simulink subsystem "mesh_assembly"  (R2021a)
settings: Solver=VariableStepAuto  StartTime=0.0  StopTime=10.0  RelTol=1e-3
undefined symbols (not defined in the file): dnm, knm, X, Y, Z
libraries: sm_lib x110, mesh_assembly_library x15
(part 3 of 4)

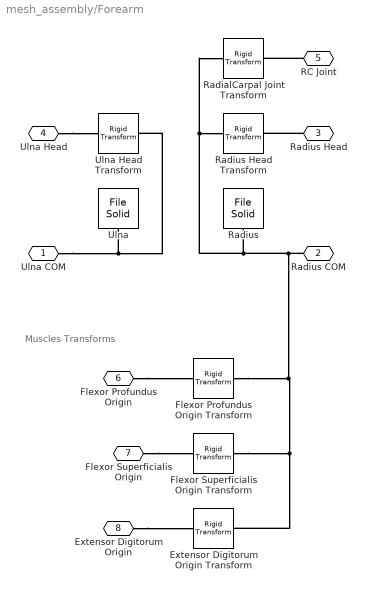
== system mesh_assembly/Forearm ==
  note: Muscles Transforms
  Extensor Digitorum Origin Transform : sm_lib/Frames and Transforms/Rigid Transform  TranslationMethod=Cartesian  TranslationStandardOffset=0  TranslationLengthUnit=m  TranslationStandardAxis=+Z  TranslationCartesianOffset=knm.radius.extensor_digitorum_origin(1,:)  TranslationROffset=0  TranslationROffsetUnits=m  TranslationZOffset=0  TranslationZOffsetUnits=m  TranslationThetaOffset=0  TranslationThetaOffsetUnits=deg  RotationMethod=RotationSequence  RotationAngleUnits=deg  RotationStandardAxis=+Z  RotationAngle=0.0  RotationArbitraryAxis=[0 0 1]  FollAlignAxisA=+X  BaseAlignAxisA=+Y  FollAlignAxisB=+Y  BaseAlignAxisB=+Z  RotationSequenceAxes=FollowerAxes  RotationSequence=XYZ  RotationSequenceAngles=knm.radius.extensor_digitorum_origin(2,:)  RotationSequenceAnglesUnits=deg  RotationMatrix=[1 0 0; 0 1 0; 0 0 1]
  Flexor Profundus Origin Transform : sm_lib/Frames and Transforms/Rigid Transform  TranslationMethod=Cartesian  TranslationStandardOffset=0  TranslationLengthUnit=m  TranslationStandardAxis=+Z  TranslationCartesianOffset=knm.radius.flexor_profundus_origin(1,:)  TranslationROffset=0  TranslationROffsetUnits=m  TranslationZOffset=0  TranslationZOffsetUnits=m  TranslationThetaOffset=0  TranslationThetaOffsetUnits=deg  RotationMethod=RotationSequence  RotationAngleUnits=deg  RotationStandardAxis=+Z  RotationAngle=0.0  RotationArbitraryAxis=[0 0 1]  FollAlignAxisA=+X  BaseAlignAxisA=+Y  FollAlignAxisB=+Y  BaseAlignAxisB=+Z  RotationSequenceAxes=FollowerAxes  RotationSequence=XYZ  RotationSequenceAngles=knm.radius.flexor_profundus_origin(2,:)  RotationSequenceAnglesUnits=deg  RotationMatrix=[1 0 0; 0 1 0; 0 0 1]
  Flexor Superficialis Origin Transform : sm_lib/Frames and Transforms/Rigid Transform  TranslationMethod=Cartesian  TranslationStandardOffset=0  TranslationLengthUnit=m  TranslationStandardAxis=+Z  TranslationCartesianOffset=knm.radius.flexor_superficialis_origin(1,:)  TranslationROffset=0  TranslationROffsetUnits=m  TranslationZOffset=0  TranslationZOffsetUnits=m  TranslationThetaOffset=0  TranslationThetaOffsetUnits=deg  RotationMethod=RotationSequence  RotationAngleUnits=deg  RotationStandardAxis=+Z  RotationAngle=0.0  RotationArbitraryAxis=[0 0 1]  FollAlignAxisA=+X  BaseAlignAxisA=+Y  FollAlignAxisB=+Y  BaseAlignAxisB=+Z  RotationSequenceAxes=FollowerAxes  RotationSequence=XYZ  RotationSequenceAngles=knm.radius.flexor_superficialis_origin(2,:)  RotationSequenceAnglesUnits=deg  RotationMatrix=[1 0 0; 0 1 0; 0 0 1]
  RadialCarpal Joint Transform : sm_lib/Frames and Transforms/Rigid Transform  TranslationMethod=Cartesian  TranslationStandardOffset=0  TranslationLengthUnit=m  TranslationStandardAxis=+Z  TranslationCartesianOffset=knm.radius.rc_joint_transform(1, :)  TranslationROffset=0  TranslationROffsetUnits=m  TranslationZOffset=0  TranslationZOffsetUnits=m  TranslationThetaOffset=0  TranslationThetaOffsetUnits=deg  RotationMethod=RotationSequence  RotationAngleUnits=deg  RotationStandardAxis=+Z  RotationAngle=0.0  RotationArbitraryAxis=[0 0 1]  FollAlignAxisA=+X  BaseAlignAxisA=+Y  FollAlignAxisB=+Y  BaseAlignAxisB=+Z  RotationSequenceAxes=FollowerAxes  RotationSequence=XYZ  RotationSequenceAngles=knm.radius.rc_joint_transform(2, :)  RotationSequenceAnglesUnits=deg  RotationMatrix=[1 0 0; 0 1 0; 0 0 1]
  Radius : sm_lib/Body Elements/File Solid  ExtGeomFileName=C:\Users\Daniel Adejumo\Documents\MATLAB\DARM\Geometry Models and FEA\Models\Skeleton Scan\Right Hand\Radius.obj  UnitType=Custom  ExtGeomFileUnits=mm  StepReaderType=HEX  ExportConvexHullGeometry=off  InertiaType=CalculateFromGeometry  Mass=1  MassUnits=kg  CenterOfMass=[0 0 0]  CenterOfMassUnits=m  MomentsOfInertia=[1 1 1]  MomentsOfInertiaUnits=kg*m^2  ProductsOfInertia=[0 0 0]  ProductsOfInertiaUnits=kg*m^2  BasedOnType=Density  Density=dnm.link_density  DensityUnits=kg/m^3  DoExposeReferenceFrame=on  SerializedFrames=<Frames><Frame><Id>Frame1</Id><Value><Name>COM</Name><Origin><Source>CenterOfMassFrame</Source><FeatureName></FeatureName></Origin><PrimaryAxis><DefinedDirection>+Z</DefinedDirection><Source>ReferenceFrame</Source><SourceDirection>-Z</SourceDirection><FeatureName></FeatureName></PrimaryAxis><SecondaryAxis><DefinedDirection>+X</DefinedDirection><Source>ReferenceFrame</Source><SourceDirection>-Y</SourceDirection><FeatureName></FeatureName></SecondaryAxis></Value></Frame></Frames>  GraphicType=FromGeometry  MarkerShape=Sphere  MarkerSize=10  GraphicVisPropType=SimpleVisualProperties  GraphicDiffuseColor=[0.5 0.5 0.5]  GraphicSpecularColor=[0.5 0.5 0.5 1.0]  GraphicAmbientColor=[0.15 0.15 0.15 1.0]  GraphicEmissiveColor=[0.0 0.0 0.0 1.0]  GraphicShininess=75  GraphicOpacity=1.0
  Radius Head Transform : sm_lib/Frames and Transforms/Rigid Transform  TranslationMethod=Cartesian  TranslationStandardOffset=0  TranslationLengthUnit=m  TranslationStandardAxis=+Z  TranslationCartesianOffset=knm.radius.head_transform(1, :)  TranslationROffset=0  TranslationROffsetUnits=m  TranslationZOffset=0  TranslationZOffsetUnits=m  TranslationThetaOffset=0  TranslationThetaOffsetUnits=deg  RotationMethod=RotationSequence  RotationAngleUnits=deg  RotationStandardAxis=+Z  RotationAngle=0.0  RotationArbitraryAxis=[0 0 1]  FollAlignAxisA=+X  BaseAlignAxisA=+Y  FollAlignAxisB=+Y  BaseAlignAxisB=+Z  RotationSequenceAxes=FollowerAxes  RotationSequence=XYZ  RotationSequenceAngles=knm.radius.head_transform(2, :)  RotationSequenceAnglesUnits=deg  RotationMatrix=[1 0 0; 0 1 0; 0 0 1]
  Ulna : sm_lib/Body Elements/File Solid  ExtGeomFileName=C:\Users\Daniel Adejumo\Documents\MATLAB\DARM\Geometry Models and FEA\Models\Skeleton Scan\Right Hand\Ulna.obj  UnitType=Custom  ExtGeomFileUnits=mm  StepReaderType=HEX  ExportConvexHullGeometry=off  InertiaType=CalculateFromGeometry  Mass=1  MassUnits=kg  CenterOfMass=[0 0 0]  CenterOfMassUnits=m  MomentsOfInertia=[1 1 1]  MomentsOfInertiaUnits=kg*m^2  ProductsOfInertia=[0 0 0]  ProductsOfInertiaUnits=kg*m^2  BasedOnType=Density  Density=dnm.link_density  DensityUnits=kg/m^3  DoExposeReferenceFrame=on  SerializedFrames=<Frames><Frame><Id>Frame1</Id><Value><Name>COM</Name><Origin><Source>CenterOfMassFrame</Source><FeatureName></FeatureName></Origin><PrimaryAxis><DefinedDirection>+Z</DefinedDirection><Source>ReferenceFrame</Source><SourceDirection>-Z</SourceDirection><FeatureName></FeatureName></PrimaryAxis><SecondaryAxis><DefinedDirection>+X</DefinedDirection><Source>ReferenceFrame</Source><SourceDirection>-Y</SourceDirection><FeatureName></FeatureName></SecondaryAxis></Value></Frame></Frames>  GraphicType=FromGeometry  MarkerShape=Sphere  MarkerSize=10  GraphicVisPropType=SimpleVisualProperties  GraphicDiffuseColor=[0.5 0.5 0.5]  GraphicSpecularColor=[0.5 0.5 0.5 1.0]  GraphicAmbientColor=[0.15 0.15 0.15 1.0]  GraphicEmissiveColor=[0.0 0.0 0.0 1.0]  GraphicShininess=75  GraphicOpacity=1.0
  Ulna Head Transform : sm_lib/Frames and Transforms/Rigid Transform  TranslationMethod=Cartesian  TranslationStandardOffset=0  TranslationLengthUnit=m  TranslationStandardAxis=+Z  TranslationCartesianOffset=knm.ulna.head_transform(1, :)  TranslationROffset=0  TranslationROffsetUnits=m  TranslationZOffset=0  TranslationZOffsetUnits=m  TranslationThetaOffset=0  TranslationThetaOffsetUnits=deg  RotationMethod=RotationSequence  RotationAngleUnits=deg  RotationStandardAxis=+Z  RotationAngle=0.0  RotationArbitraryAxis=[0 0 1]  FollAlignAxisA=+X  BaseAlignAxisA=+Y  FollAlignAxisB=+Y  BaseAlignAxisB=+Z  RotationSequenceAxes=FollowerAxes  RotationSequence=XYZ  RotationSequenceAngles=knm.ulna.head_transform(2, :)  RotationSequenceAnglesUnits=deg  RotationMatrix=[1 0 0; 0 1 0; 0 0 1]
  Ulna COM : PMIOPort  Side=Left
  Radius COM : PMIOPort  Port=2  Side=Left
  Radius Head : PMIOPort  Port=3  Side=Left
  Ulna Head : PMIOPort  Port=4  Side=Left
  RC Joint : PMIOPort  Port=5  Side=Right
  Flexor Profundus Origin : PMIOPort  Port=6  Side=Left
  Flexor Superficialis Origin : PMIOPort  Port=7  Side=Left
  Extensor Digitorum Origin : PMIOPort  Port=8  Side=Left
  connections:
  Flexor Profundus Origin/RConn1 -- Flexor Profundus Origin Transform/RConn1
  Extensor Digitorum Origin/RConn1 -- Extensor Digitorum Origin Transform/RConn1
  Flexor Superficialis Origin/RConn1 -- Flexor Superficialis Origin Transform/RConn1
  Flexor Profundus Origin Transform/LConn1 -- Flexor Superficialis Origin Transform/LConn1 -- Extensor Digitorum Origin Transform/LConn1 -- Radius COM/RConn1 -- RadialCarpal Joint Transform/LConn1 -- Radius Head Transform/LConn1 -- Radius/LConn1
  Ulna COM/RConn1 -- Ulna/LConn1 -- Ulna Head Transform/LConn1
  RC Joint/RConn1 -- RadialCarpal Joint Transform/RConn1
  Radius Head/RConn1 -- Radius Head Transform/RConn1
  Ulna Head/RConn1 -- Ulna Head Transform/RConn1

== system mesh_assembly/RC Primitive Joint ==
  Universal Joint : sm_lib/Joints/Universal Joint  JointMode=Normal  SenseConstraintForce=off  SenseConstraintForceX=off  SenseConstraintForceY=off  SenseConstraintForceZ=off  SenseConstraintTorque=off  SenseConstraintTorqueX=off  SenseConstraintTorqueY=off  SenseConstraintTorqueZ=off  SenseTotalForce=off  SenseTotalForceX=off  SenseTotalForceY=off  SenseTotalForceZ=off  SenseTotalTorque=off  SenseTotalTorqueX=off  SenseTotalTorqueY=off  SenseTotalTorqueZ=off  CompositeWrenchDir=FollowerOnBase  CompositeWrenchFrame=BaseFrame  RxEquilibriumPosition=0  RxEquilibriumPositionUnits=deg  RxSpringStiffness=stiffness  RxSpringStiffnessUnits=N*m/deg  RxDampingCoefficient=damping  RxDampingCoefficientUnits=N*m/(deg/s)  RxTorqueActuationMode=NoTorque  RxMotionActuationMode=ComputedMotion  RxSensePosition=off  RxSenseVelocity=off  RxSenseAcceleration=off  RxSenseTorqueForce=off  RxSenseLowerLimitTorqueForce=off  RxSenseUpperLimitTorqueForce=off  RxLowerLimitSpecify=on  RxLowerLimitBound=x_limits(1)  RxLowerLimitBoundUnits=deg  RxLowerLimitStiffness=1e4  RxLowerLimitStiffnessUnits=N*m/deg  RxLowerLimitDamping=10  RxLowerLimitDampingUnits=N*m/(deg/s)  RxLowerLimitTransitionRegionWidth=0.1  RxLowerLimitTransitionRegionWidthUnits=deg  RxUpperLimitSpecify=on  RxUpperLimitBound=x_limits(2)  RxUpperLimitBoundUnits=deg  RxUpperLimitStiffness=1e4  RxUpperLimitStiffnessUnits=N*m/deg  RxUpperLimitDamping=10  RxUpperLimitDampingUnits=N*m/(deg/s)  RxUpperLimitTransitionRegionWidth=0.1  RxUpperLimitTransitionRegionWidthUnits=deg  RxPositionTargetSpecify=on  RxPositionTargetPriority=High  RxPositionTargetValue=x_initial_position  RxPositionTargetValueUnits=deg  RxVelocityTargetSpecify=off  RxVelocityTargetPriority=High  RxVelocityTargetValue=0  RxVelocityTargetValueUnits=deg/s  RyEquilibriumPosition=0  RyEquilibriumPositionUnits=deg  RySpringStiffness=stiffness  RySpringStiffnessUnits=N*m/deg  RyDampingCoefficient=damping  RyDampingCoefficientUnits=N*m/(deg/s)  RyTorqueActuationMode=NoTorque  RyMotionActuationMode=ComputedMotion  RySensePosition=off  RySenseVelocity=off  RySenseAcceleration=off  RySenseTorqueForce=off  RySenseLowerLimitTorqueForce=off  RySenseUpperLimitTorqueForce=off  RyLowerLimitSpecify=on  RyLowerLimitBound=y_limits(1)  RyLowerLimitBoundUnits=deg  RyLowerLimitStiffness=1e4  RyLowerLimitStiffnessUnits=N*m/deg  RyLowerLimitDamping=10  RyLowerLimitDampingUnits=N*m/(deg/s)  RyLowerLimitTransitionRegionWidth=0.1  RyLowerLimitTransitionRegionWidthUnits=deg  RyUpperLimitSpecify=on  RyUpperLimitBound=y_limits(2)  RyUpperLimitBoundUnits=deg  RyUpperLimitStiffness=1e4  RyUpperLimitStiffnessUnits=N*m/deg  RyUpperLimitDamping=10  RyUpperLimitDampingUnits=N*m/(deg/s)  RyUpperLimitTransitionRegionWidth=0.1  RyUpperLimitTransitionRegionWidthUnits=deg  RyPositionTargetSpecify=on  RyPositionTargetPriority=High  RyPositionTargetValue=y_initial_position  RyPositionTargetValueUnits=deg  RyVelocityTargetSpecify=off  RyVelocityTargetPriority=High  RyVelocityTargetValue=0  RyVelocityTargetValueUnits=deg/s
  X Axis Viz Transform : sm_lib/Frames and Transforms/Rigid Transform  TranslationMethod=None  TranslationStandardOffset=0  TranslationLengthUnit=m  TranslationStandardAxis=+Z  TranslationCartesianOffset=[0 0 0]  TranslationROffset=0  TranslationROffsetUnits=m  TranslationZOffset=0  TranslationZOffsetUnits=m  TranslationThetaOffset=0  TranslationThetaOffsetUnits=deg  RotationMethod=AlignedAxes  RotationAngleUnits=deg  RotationStandardAxis=+Z  RotationAngle=0.0  RotationArbitraryAxis=[0 0 1]  FollAlignAxisA=+Z  BaseAlignAxisA=+X  FollAlignAxisB=+X  BaseAlignAxisB=+Z  RotationSequenceAxes=FollowerAxes  RotationSequence=XYX  RotationSequenceAngles=[0 0 0]  RotationSequenceAnglesUnits=deg  RotationMatrix=[1 0 0; 0 1 0; 0 0 1]
  X Viz Cylinder : sm_lib/Body Elements/Revolved Solid  GraphicAmbientColor=[0.15 0.15 0.15 1.0]  BasedOnType=Mass  CenterOfMass=[0 0 0]  CenterOfMassUnits=m  GraphicDiffuseColor=x_color  ExportConvexHullGeometry=off  Density=1000  DensityUnits=kg/m^3  DoExposeReferenceFrame=on  GraphicEmissiveColor=[0.0 0.0 0.0 1.0]  ExportEntireGeometry=off  SerializedFrames=<Frames/>  MarkerShape=Sphere  MarkerSize=10  GraphicType=FromGeometry  InertiaType=CalculateFromGeometry  Mass=0  MassUnits=kg  MomentsOfInertia=[1 1 1]  MomentsOfInertiaUnits=kg*m^2  GraphicOpacity=x_opacity  ProductsOfInertia=[0 0 0]  ProductsOfInertiaUnits=kg*m^2  RevolutionCrossSection=|  RevolutionCrossSectionUnits=m  RevolutionAngle=180  RevolutionAngleUnits=deg  RevolutionExtent=Full  GraphicShininess=75  GraphicSpecularColor=[0.5 0.5 0.5 1.0]  GraphicVisPropType=SimpleVisualProperties
      | [x_radius, x_length/2;
      |  x_radius, -x_length/2;
      |  x_radius+thickness, -x_length/2;
      |  x_radius+thickness, x_length/2]
  Y Axis Viz Transform : sm_lib/Frames and Transforms/Rigid Transform  TranslationMethod=None  TranslationStandardOffset=0  TranslationLengthUnit=m  TranslationStandardAxis=+Z  TranslationCartesianOffset=[0 0 0]  TranslationROffset=0  TranslationROffsetUnits=m  TranslationZOffset=0  TranslationZOffsetUnits=m  TranslationThetaOffset=0  TranslationThetaOffsetUnits=deg  RotationMethod=AlignedAxes  RotationAngleUnits=deg  RotationStandardAxis=+Z  RotationAngle=0.0  RotationArbitraryAxis=[0 0 1]  FollAlignAxisA=+Z  BaseAlignAxisA=+Y  FollAlignAxisB=+X  BaseAlignAxisB=+Z  RotationSequenceAxes=FollowerAxes  RotationSequence=XYX  RotationSequenceAngles=[0 0 0]  RotationSequenceAnglesUnits=deg  RotationMatrix=[1 0 0; 0 1 0; 0 0 1]
  Y Viz Cylinder : sm_lib/Body Elements/Revolved Solid  GraphicAmbientColor=[0.15 0.15 0.15 1.0]  BasedOnType=Mass  CenterOfMass=[0 0 0]  CenterOfMassUnits=m  GraphicDiffuseColor=y_color  ExportConvexHullGeometry=off  Density=1000  DensityUnits=kg/m^3  DoExposeReferenceFrame=on  GraphicEmissiveColor=[0.0 0.0 0.0 1.0]  ExportEntireGeometry=off  SerializedFrames=<Frames/>  MarkerShape=Sphere  MarkerSize=10  GraphicType=FromGeometry  InertiaType=CalculateFromGeometry  Mass=0  MassUnits=kg  MomentsOfInertia=[1 1 1]  MomentsOfInertiaUnits=kg*m^2  GraphicOpacity=y_opacity  ProductsOfInertia=[0 0 0]  ProductsOfInertiaUnits=kg*m^2  RevolutionCrossSection=|  RevolutionCrossSectionUnits=m  RevolutionAngle=180  RevolutionAngleUnits=deg  RevolutionExtent=Full  GraphicShininess=75  GraphicSpecularColor=[0.5 0.5 0.5 1.0]  GraphicVisPropType=SimpleVisualProperties
      | [y_radius, y_length/2;
      |  y_radius, -y_length/2;
      |  y_radius+thickness, -y_length/2;
      |  y_radius+thickness, y_length/2]
  F : PMIOPort  Side=Right
  B : PMIOPort  Port=2  Side=Left
  connections:
  Y Viz Cylinder/RConn1 -- Y Axis Viz Transform/RConn1
  X Axis Viz Transform/RConn1 -- X Viz Cylinder/RConn1
  Y Axis Viz Transform/LConn1 -- Universal Joint/RConn1 -- F/RConn1
  X Axis Viz Transform/LConn1 -- B/RConn1 -- Universal Joint/LConn1

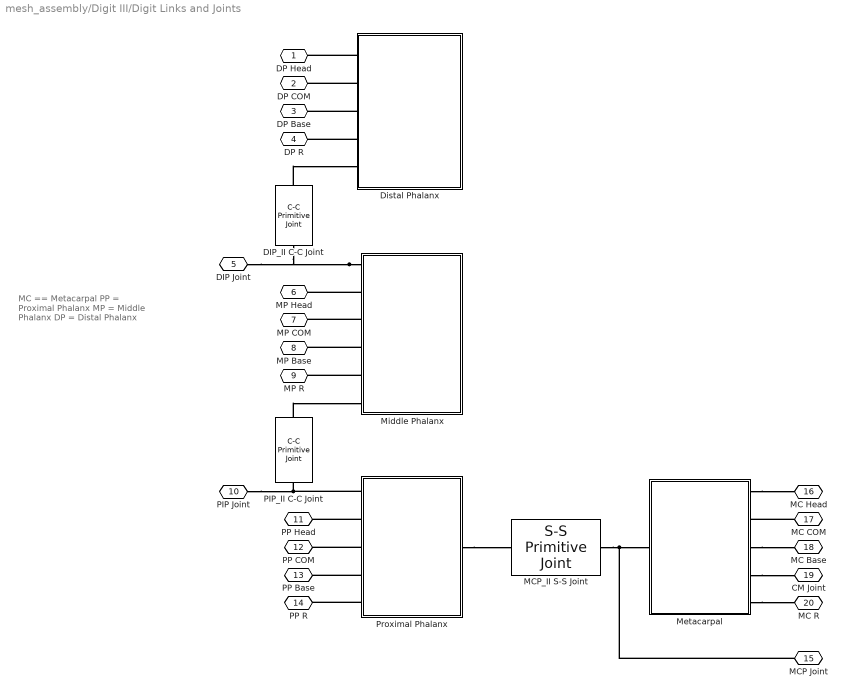
== system mesh_assembly/Digit III/Digit Links and Joints ==
  note: MC == Metacarpal
      | PP = Proximal Phalanx
      | MP = Middle Phalanx
      | DP = Distal Phalanx
  DIP_II C-C Joint : mesh_assembly_library/C-C Primitive Joint  stiffness=0  damping=0  lower_limit=-90  upper_limit=90  initial_position=0  radius=dip_viz_radius  length=dip_viz_length  thickness=dip_viz_thickness  color=dip_viz_color  opacity=dip_viz_opacity
  Distal Phalanx : Subsystem
  MCP_II S-S Joint : mesh_assembly_library/S-S Primitive Joint  stiffness=0  damping=0  x_limits=[-90 90]  y_limits=[-90 90]  x_initial_position=0  y_initial_position=0  radius=mcp_viz_radius  color=mcp_viz_color  opacity=mcp_viz_opacity
  Metacarpal : Subsystem
  Middle Phalanx : Subsystem
  PIP_II C-C Joint : mesh_assembly_library/C-C Primitive Joint  stiffness=0  damping=0  lower_limit=-90  upper_limit=90  initial_position=0  radius=pip_viz_radius  length=pip_viz_length  thickness=pip_viz_thickness  color=pip_viz_color  opacity=pip_viz_opacity
  Proximal Phalanx : Subsystem
  DP Head : PMIOPort  Side=Left
  DP COM : PMIOPort  Port=2  Side=Left
  DP Base : PMIOPort  Port=3  Side=Left
  DP R : PMIOPort  Port=4  Side=Left
  DIP Joint : PMIOPort  Port=5  Side=Left
  MP Head : PMIOPort  Port=6  Side=Left
  MP COM : PMIOPort  Port=7  Side=Left
  MP Base : PMIOPort  Port=8  Side=Left
  MP R : PMIOPort  Port=9  Side=Left
  PIP Joint : PMIOPort  Port=10  Side=Left
  PP Head : PMIOPort  Port=11  Side=Left
  PP COM : PMIOPort  Port=12  Side=Left
  PP Base : PMIOPort  Port=13  Side=Left
  PP R : PMIOPort  Port=14  Side=Left
  MCP Joint : PMIOPort  Port=15  Side=Left
  MC Head : PMIOPort  Port=16  Side=Left
  MC COM : PMIOPort  Port=17  Side=Left
  MC Base : PMIOPort  Port=18  Side=Left
  CM Joint : PMIOPort  Port=19  Side=Left
  MC R : PMIOPort  Port=20  Side=Left
  connections:
  Proximal Phalanx/LConn5 -- PP R/RConn1
  Proximal Phalanx/LConn4 -- PP Base/RConn1
  Proximal Phalanx/LConn2 -- PP Head/RConn1
  Distal Phalanx/LConn1 -- DP Head/RConn1
  Distal Phalanx/LConn2 -- DP COM/RConn1
  Metacarpal/RConn5 -- MC R/RConn1
  Metacarpal/RConn1 -- MC Head/RConn1
  Metacarpal/RConn4 -- CM Joint/RConn1
  Metacarpal/RConn3 -- MC Base/RConn1
  Middle Phalanx/LConn4 -- MP Base/RConn1
  Middle Phalanx/LConn2 -- MP Head/RConn1
  PIP_II C-C Joint/RConn1 -- Middle Phalanx/LConn6
  Distal Phalanx/LConn4 -- DP R/RConn1
  MCP Joint/RConn1 -- MCP_II S-S Joint/LConn1 -- Metacarpal/LConn1
  Middle Phalanx/LConn3 -- MP COM/RConn1
  Proximal Phalanx/LConn3 -- PP COM/RConn1
  Middle Phalanx/LConn1 -- DIP_II C-C Joint/LConn1 -- DIP Joint/RConn1
  Middle Phalanx/LConn5 -- MP R/RConn1
  Distal Phalanx/LConn3 -- DP Base/RConn1
  Proximal Phalanx/RConn1 -- MCP_II S-S Joint/RConn1
  PIP Joint/RConn1 -- Proximal Phalanx/LConn1 -- PIP_II C-C Joint/LConn1
  DIP_II C-C Joint/RConn1 -- Distal Phalanx/LConn5
  MC COM/RConn1 -- Metacarpal/RConn2

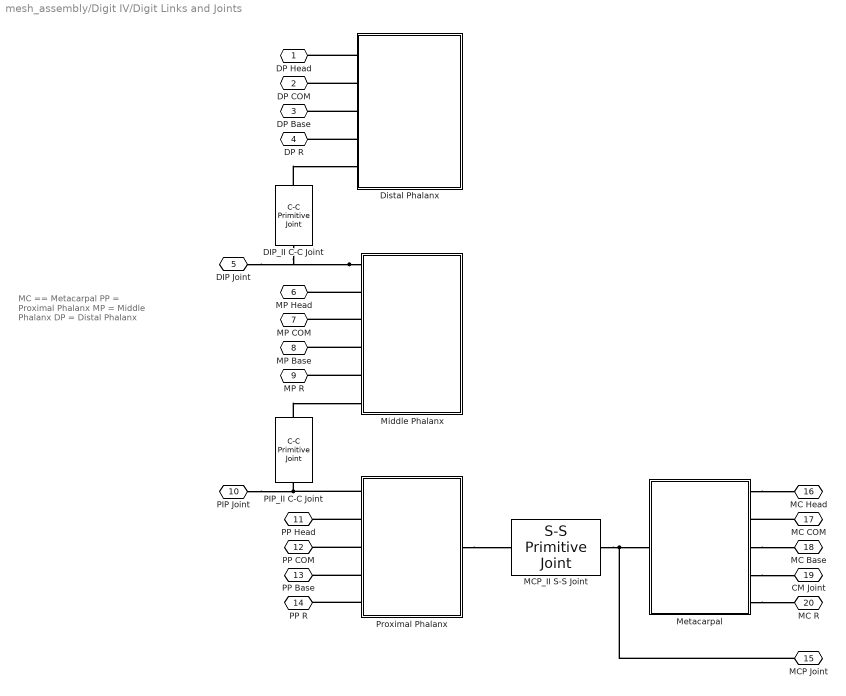
== system mesh_assembly/Digit IV/Digit Links and Joints ==
  note: MC == Metacarpal
      | PP = Proximal Phalanx
      | MP = Middle Phalanx
      | DP = Distal Phalanx
  DIP_II C-C Joint : mesh_assembly_library/C-C Primitive Joint  stiffness=0  damping=0  lower_limit=-90  upper_limit=90  initial_position=0  radius=dip_viz_radius  length=dip_viz_length  thickness=dip_viz_thickness  color=dip_viz_color  opacity=dip_viz_opacity
  Distal Phalanx : Subsystem
  MCP_II S-S Joint : mesh_assembly_library/S-S Primitive Joint  stiffness=0  damping=0  x_limits=[-90 90]  y_limits=[-90 90]  x_initial_position=0  y_initial_position=0  radius=mcp_viz_radius  color=mcp_viz_color  opacity=mcp_viz_opacity
  Metacarpal : Subsystem
  Middle Phalanx : Subsystem
  PIP_II C-C Joint : mesh_assembly_library/C-C Primitive Joint  stiffness=0  damping=0  lower_limit=-90  upper_limit=90  initial_position=0  radius=pip_viz_radius  length=pip_viz_length  thickness=pip_viz_thickness  color=pip_viz_color  opacity=pip_viz_opacity
  Proximal Phalanx : Subsystem
  DP Head : PMIOPort  Side=Left
  DP COM : PMIOPort  Port=2  Side=Left
  DP Base : PMIOPort  Port=3  Side=Left
  DP R : PMIOPort  Port=4  Side=Left
  DIP Joint : PMIOPort  Port=5  Side=Left
  MP Head : PMIOPort  Port=6  Side=Left
  MP COM : PMIOPort  Port=7  Side=Left
  MP Base : PMIOPort  Port=8  Side=Left
  MP R : PMIOPort  Port=9  Side=Left
  PIP Joint : PMIOPort  Port=10  Side=Left
  PP Head : PMIOPort  Port=11  Side=Left
  PP COM : PMIOPort  Port=12  Side=Left
  PP Base : PMIOPort  Port=13  Side=Left
  PP R : PMIOPort  Port=14  Side=Left
  MCP Joint : PMIOPort  Port=15  Side=Left
  MC Head : PMIOPort  Port=16  Side=Left
  MC COM : PMIOPort  Port=17  Side=Left
  MC Base : PMIOPort  Port=18  Side=Left
  CM Joint : PMIOPort  Port=19  Side=Left
  MC R : PMIOPort  Port=20  Side=Left
  connections:
  Proximal Phalanx/LConn5 -- PP R/RConn1
  Proximal Phalanx/LConn4 -- PP Base/RConn1
  Proximal Phalanx/LConn2 -- PP Head/RConn1
  Distal Phalanx/LConn1 -- DP Head/RConn1
  Distal Phalanx/LConn2 -- DP COM/RConn1
  Metacarpal/RConn5 -- MC R/RConn1
  Metacarpal/RConn1 -- MC Head/RConn1
  Metacarpal/RConn4 -- CM Joint/RConn1
  Metacarpal/RConn3 -- MC Base/RConn1
  Middle Phalanx/LConn4 -- MP Base/RConn1
  Middle Phalanx/LConn2 -- MP Head/RConn1
  PIP_II C-C Joint/RConn1 -- Middle Phalanx/LConn6
  Distal Phalanx/LConn4 -- DP R/RConn1
  MCP Joint/RConn1 -- MCP_II S-S Joint/LConn1 -- Metacarpal/LConn1
  Middle Phalanx/LConn3 -- MP COM/RConn1
  Proximal Phalanx/LConn3 -- PP COM/RConn1
  Middle Phalanx/LConn1 -- DIP_II C-C Joint/LConn1 -- DIP Joint/RConn1
  Middle Phalanx/LConn5 -- MP R/RConn1
  Distal Phalanx/LConn3 -- DP Base/RConn1
  Proximal Phalanx/RConn1 -- MCP_II S-S Joint/RConn1
  PIP Joint/RConn1 -- Proximal Phalanx/LConn1 -- PIP_II C-C Joint/LConn1
  DIP_II C-C Joint/RConn1 -- Distal Phalanx/LConn5
  MC COM/RConn1 -- Metacarpal/RConn2

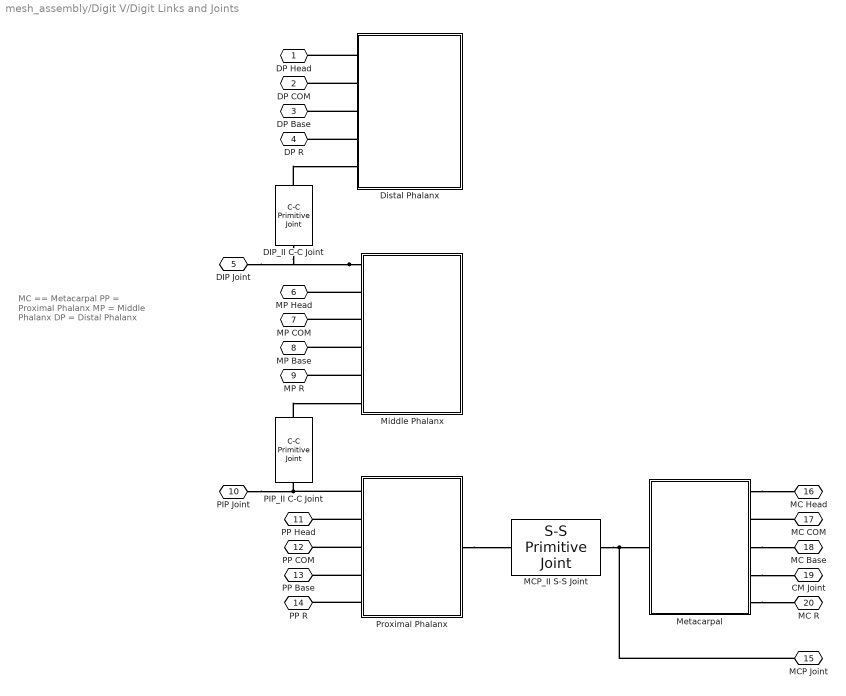
== system mesh_assembly/Digit V/Digit Links and Joints ==
  note: MC == Metacarpal
      | PP = Proximal Phalanx
      | MP = Middle Phalanx
      | DP = Distal Phalanx
  DIP_II C-C Joint : mesh_assembly_library/C-C Primitive Joint  stiffness=0  damping=0  lower_limit=-90  upper_limit=90  initial_position=0  radius=dip_viz_radius  length=dip_viz_length  thickness=dip_viz_thickness  color=dip_viz_color  opacity=dip_viz_opacity
  Distal Phalanx : Subsystem
  MCP_II S-S Joint : mesh_assembly_library/S-S Primitive Joint  stiffness=0  damping=0  x_limits=[-90 90]  y_limits=[-90 90]  x_initial_position=0  y_initial_position=0  radius=mcp_viz_radius  color=mcp_viz_color  opacity=mcp_viz_opacity
  Metacarpal : Subsystem
  Middle Phalanx : Subsystem
  PIP_II C-C Joint : mesh_assembly_library/C-C Primitive Joint  stiffness=0  damping=0  lower_limit=-90  upper_limit=90  initial_position=0  radius=pip_viz_radius  length=pip_viz_length  thickness=pip_viz_thickness  color=pip_viz_color  opacity=pip_viz_opacity
  Proximal Phalanx : Subsystem
  DP Head : PMIOPort  Side=Left
  DP COM : PMIOPort  Port=2  Side=Left
  DP Base : PMIOPort  Port=3  Side=Left
  DP R : PMIOPort  Port=4  Side=Left
  DIP Joint : PMIOPort  Port=5  Side=Left
  MP Head : PMIOPort  Port=6  Side=Left
  MP COM : PMIOPort  Port=7  Side=Left
  MP Base : PMIOPort  Port=8  Side=Left
  MP R : PMIOPort  Port=9  Side=Left
  PIP Joint : PMIOPort  Port=10  Side=Left
  PP Head : PMIOPort  Port=11  Side=Left
  PP COM : PMIOPort  Port=12  Side=Left
  PP Base : PMIOPort  Port=13  Side=Left
  PP R : PMIOPort  Port=14  Side=Left
  MCP Joint : PMIOPort  Port=15  Side=Left
  MC Head : PMIOPort  Port=16  Side=Left
  MC COM : PMIOPort  Port=17  Side=Left
  MC Base : PMIOPort  Port=18  Side=Left
  CM Joint : PMIOPort  Port=19  Side=Left
  MC R : PMIOPort  Port=20  Side=Left
  connections:
  Proximal Phalanx/LConn5 -- PP R/RConn1
  Proximal Phalanx/LConn4 -- PP Base/RConn1
  Proximal Phalanx/LConn2 -- PP Head/RConn1
  Distal Phalanx/LConn1 -- DP Head/RConn1
  Distal Phalanx/LConn2 -- DP COM/RConn1
  Metacarpal/RConn5 -- MC R/RConn1
  Metacarpal/RConn1 -- MC Head/RConn1
  Metacarpal/RConn4 -- CM Joint/RConn1
  Metacarpal/RConn3 -- MC Base/RConn1
  Middle Phalanx/LConn4 -- MP Base/RConn1
  Middle Phalanx/LConn2 -- MP Head/RConn1
  PIP_II C-C Joint/RConn1 -- Middle Phalanx/LConn6
  Distal Phalanx/LConn4 -- DP R/RConn1
  MCP Joint/RConn1 -- MCP_II S-S Joint/LConn1 -- Metacarpal/LConn1
  Middle Phalanx/LConn3 -- MP COM/RConn1
  Proximal Phalanx/LConn3 -- PP COM/RConn1
  Middle Phalanx/LConn1 -- DIP_II C-C Joint/LConn1 -- DIP Joint/RConn1
  Middle Phalanx/LConn5 -- MP R/RConn1
  Distal Phalanx/LConn3 -- DP Base/RConn1
  Proximal Phalanx/RConn1 -- MCP_II S-S Joint/RConn1
  PIP Joint/RConn1 -- Proximal Phalanx/LConn1 -- PIP_II C-C Joint/LConn1
  DIP_II C-C Joint/RConn1 -- Distal Phalanx/LConn5
  MC COM/RConn1 -- Metacarpal/RConn2

== system mesh_assembly/Digit III/Digit Links and Joints/Distal Phalanx ==
  Base Transform : sm_lib/Frames and Transforms/Rigid Transform  TranslationMethod=Cartesian  TranslationStandardOffset=0  TranslationLengthUnit=m  TranslationStandardAxis=+Z  TranslationCartesianOffset=distal_phalanx_base(1, :)  TranslationROffset=0  TranslationROffsetUnits=m  TranslationZOffset=0  TranslationZOffsetUnits=m  TranslationThetaOffset=0  TranslationThetaOffsetUnits=deg  RotationMethod=RotationSequence  RotationAngleUnits=deg  RotationStandardAxis=+Z  RotationAngle=0.0  RotationArbitraryAxis=[0 0 1]  FollAlignAxisA=+X  BaseAlignAxisA=+Y  FollAlignAxisB=+Y  BaseAlignAxisB=+Z  RotationSequenceAxes=FollowerAxes  RotationSequence=XYZ  RotationSequenceAngles=distal_phalanx_base(2, :)  RotationSequenceAnglesUnits=deg  RotationMatrix=[1 0 0; 0 1 0; 0 0 1]
  DIP Joint Transform : sm_lib/Frames and Transforms/Rigid Transform  TranslationMethod=Cartesian  TranslationStandardOffset=0  TranslationLengthUnit=m  TranslationStandardAxis=+Z  TranslationCartesianOffset=distal_phalanx_dip_joint(1, :)  TranslationROffset=0  TranslationROffsetUnits=m  TranslationZOffset=0  TranslationZOffsetUnits=m  TranslationThetaOffset=0  TranslationThetaOffsetUnits=deg  RotationMethod=RotationSequence  RotationAngleUnits=deg  RotationStandardAxis=+Z  RotationAngle=0.0  RotationArbitraryAxis=[0 0 1]  FollAlignAxisA=+X  BaseAlignAxisA=+Y  FollAlignAxisB=+Y  BaseAlignAxisB=+Z  RotationSequenceAxes=FollowerAxes  RotationSequence=XYZ  RotationSequenceAngles=distal_phalanx_dip_joint(2, :)  RotationSequenceAnglesUnits=deg  RotationMatrix=[1 0 0; 0 1 0; 0 0 1]
  Head Transform : sm_lib/Frames and Transforms/Rigid Transform  TranslationMethod=Cartesian  TranslationStandardOffset=0  TranslationLengthUnit=m  TranslationStandardAxis=+Z  TranslationCartesianOffset=distal_phalanx_head(1, :)  TranslationROffset=0  TranslationROffsetUnits=m  TranslationZOffset=0  TranslationZOffsetUnits=m  TranslationThetaOffset=0  TranslationThetaOffsetUnits=deg  RotationMethod=RotationSequence  RotationAngleUnits=deg  RotationStandardAxis=+Z  RotationAngle=0.0  RotationArbitraryAxis=[0 0 1]  FollAlignAxisA=+X  BaseAlignAxisA=+Y  FollAlignAxisB=+Y  BaseAlignAxisB=+Z  RotationSequenceAxes=FollowerAxes  RotationSequence=XYZ  RotationSequenceAngles=distal_phalanx_head(2, :)  RotationSequenceAnglesUnits=deg  RotationMatrix=[1 0 0; 0 1 0; 0 0 1]
  Rigid Body : sm_lib/Body Elements/File Solid  ExtGeomFileName=C:\Users\Daniel Adejumo\Documents\MATLAB\DARM\Geometry Models and FEA\Models\Skeleton Scan\Right Hand\Digit III\Distal Phalanx III.obj  UnitType=Custom  ExtGeomFileUnits=mm  StepReaderType=HEX  ExportConvexHullGeometry=off  InertiaType=CalculateFromGeometry  Mass=1  MassUnits=kg  CenterOfMass=[0 0 0]  CenterOfMassUnits=m  MomentsOfInertia=[1 1 1]  MomentsOfInertiaUnits=kg*m^2  ProductsOfInertia=[0 0 0]  ProductsOfInertiaUnits=kg*m^2  BasedOnType=Density  Density=links_density  DensityUnits=kg/m^3  DoExposeReferenceFrame=on  SerializedFrames=<Frames><Frame><Id>Frame1</Id><Value><Name>COM</Name><Origin><Source>CenterOfMassFrame</Source><FeatureName></FeatureName></Origin><PrimaryAxis><DefinedDirection>+Z</DefinedDirection><Source>ReferenceFrame</Source><SourceDirection>+X</SourceDirection><FeatureName></FeatureName></PrimaryAxis><SecondaryAxis><DefinedDirection>+X</DefinedDirection><Source>ReferenceFrame</Source><SourceDirection>-Y</SourceDirection><FeatureName></FeatureName></SecondaryAxis></Value></Frame></Frames>  GraphicType=FromGeometry  MarkerShape=Sphere  MarkerSize=10  GraphicVisPropType=SimpleVisualProperties  GraphicDiffuseColor=[0.5 0.5 0.5]  GraphicSpecularColor=[0.5 0.5 0.5 1.0]  GraphicAmbientColor=[0.15 0.15 0.15 1.0]  GraphicEmissiveColor=[0.0 0.0 0.0 1.0]  GraphicShininess=75  GraphicOpacity=1.0
  Head : PMIOPort  Side=Left
  COM : PMIOPort  Port=2  Side=Left
  Base : PMIOPort  Port=3  Side=Left
  R : PMIOPort  Port=4  Side=Left
  DIP Joint : PMIOPort  Port=5  Side=Left
  connections:
  R/RConn1 -- Rigid Body/RConn1
  Head/RConn1 -- Head Transform/RConn1
  DIP Joint/RConn1 -- DIP Joint Transform/RConn1
  Base/RConn1 -- Base Transform/RConn1
  DIP Joint Transform/LConn1 -- Rigid Body/LConn1 -- Head Transform/LConn1 -- COM/RConn1 -- Base Transform/LConn1

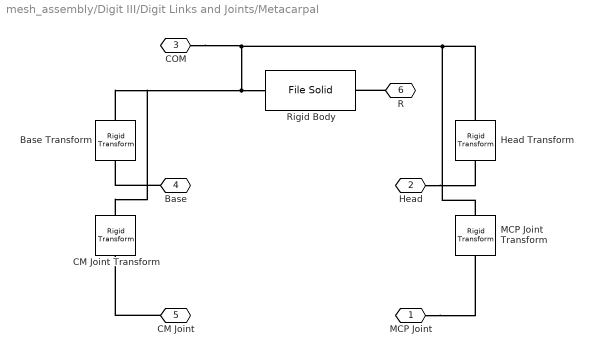
== system mesh_assembly/Digit III/Digit Links and Joints/Metacarpal ==
  Base Transform : sm_lib/Frames and Transforms/Rigid Transform  TranslationMethod=Cartesian  TranslationStandardOffset=0  TranslationLengthUnit=m  TranslationStandardAxis=+Z  TranslationCartesianOffset=metacarpal_base(1, :)  TranslationROffset=0  TranslationROffsetUnits=m  TranslationZOffset=0  TranslationZOffsetUnits=m  TranslationThetaOffset=0  TranslationThetaOffsetUnits=deg  RotationMethod=RotationSequence  RotationAngleUnits=deg  RotationStandardAxis=+Z  RotationAngle=0.0  RotationArbitraryAxis=[0 0 1]  FollAlignAxisA=+X  BaseAlignAxisA=+Y  FollAlignAxisB=+Y  BaseAlignAxisB=+Z  RotationSequenceAxes=FollowerAxes  RotationSequence=XYZ  RotationSequenceAngles=metacarpal_base(2, :)  RotationSequenceAnglesUnits=deg  RotationMatrix=[1 0 0; 0 1 0; 0 0 1]
  CM Joint Transform : sm_lib/Frames and Transforms/Rigid Transform  TranslationMethod=Cartesian  TranslationStandardOffset=0  TranslationLengthUnit=m  TranslationStandardAxis=+Z  TranslationCartesianOffset=metacarpal_cm_joint(1, :)  TranslationROffset=0  TranslationROffsetUnits=m  TranslationZOffset=0  TranslationZOffsetUnits=m  TranslationThetaOffset=0  TranslationThetaOffsetUnits=deg  RotationMethod=RotationSequence  RotationAngleUnits=deg  RotationStandardAxis=+Z  RotationAngle=0.0  RotationArbitraryAxis=[0 0 1]  FollAlignAxisA=+X  BaseAlignAxisA=+Y  FollAlignAxisB=+Y  BaseAlignAxisB=+Z  RotationSequenceAxes=FollowerAxes  RotationSequence=XYZ  RotationSequenceAngles=metacarpal_cm_joint(2, :)  RotationSequenceAnglesUnits=deg  RotationMatrix=[1 0 0; 0 1 0; 0 0 1]
  Head Transform : sm_lib/Frames and Transforms/Rigid Transform  TranslationMethod=Cartesian  TranslationStandardOffset=0  TranslationLengthUnit=m  TranslationStandardAxis=+Z  TranslationCartesianOffset=metacarpal_head(1, :)  TranslationROffset=0  TranslationROffsetUnits=m  TranslationZOffset=0  TranslationZOffsetUnits=m  TranslationThetaOffset=0  TranslationThetaOffsetUnits=deg  RotationMethod=RotationSequence  RotationAngleUnits=deg  RotationStandardAxis=+Z  RotationAngle=0.0  RotationArbitraryAxis=[0 0 1]  FollAlignAxisA=+X  BaseAlignAxisA=+Y  FollAlignAxisB=+Y  BaseAlignAxisB=+Z  RotationSequenceAxes=FollowerAxes  RotationSequence=XYZ  RotationSequenceAngles=metacarpal_head(2, :)  RotationSequenceAnglesUnits=deg  RotationMatrix=[1 0 0; 0 1 0; 0 0 1]
  MCP Joint Transform : sm_lib/Frames and Transforms/Rigid Transform  TranslationMethod=Cartesian  TranslationStandardOffset=0  TranslationLengthUnit=m  TranslationStandardAxis=+Z  TranslationCartesianOffset=metacarpal_mcp_joint(1, :)  TranslationROffset=0  TranslationROffsetUnits=m  TranslationZOffset=0  TranslationZOffsetUnits=m  TranslationThetaOffset=0  TranslationThetaOffsetUnits=deg  RotationMethod=RotationSequence  RotationAngleUnits=deg  RotationStandardAxis=+Z  RotationAngle=0.0  RotationArbitraryAxis=[0 0 1]  FollAlignAxisA=+X  BaseAlignAxisA=+Y  FollAlignAxisB=+Y  BaseAlignAxisB=+Z  RotationSequenceAxes=FollowerAxes  RotationSequence=XYZ  RotationSequenceAngles=metacarpal_mcp_joint(2, :)  RotationSequenceAnglesUnits=deg  RotationMatrix=[1 0 0; 0 1 0; 0 0 1]
  Rigid Body : sm_lib/Body Elements/File Solid  ExtGeomFileName=C:\Users\Daniel Adejumo\Documents\MATLAB\DARM\Geometry Models and FEA\Models\Skeleton Scan\Right Hand\Digit III\Metacarpal III.obj  UnitType=Custom  ExtGeomFileUnits=mm  StepReaderType=HEX  ExportConvexHullGeometry=off  InertiaType=CalculateFromGeometry  Mass=1  MassUnits=kg  CenterOfMass=[0 0 0]  CenterOfMassUnits=m  MomentsOfInertia=[1 1 1]  MomentsOfInertiaUnits=kg*m^2  ProductsOfInertia=[0 0 0]  ProductsOfInertiaUnits=kg*m^2  BasedOnType=Density  Density=links_density  DensityUnits=kg/m^3  DoExposeReferenceFrame=on  SerializedFrames=<Frames><Frame><Id>Frame1</Id><Value><Name>COM</Name><Origin><Source>CenterOfMassFrame</Source><FeatureName></FeatureName></Origin><PrimaryAxis><DefinedDirection>+Z</DefinedDirection><Source>ReferenceFrame</Source><SourceDirection>-Z</SourceDirection><FeatureName></FeatureName></PrimaryAxis><SecondaryAxis><DefinedDirection>+X</DefinedDirection><Source>ReferenceFrame</Source><SourceDirection>-Y</SourceDirection><FeatureName></FeatureName></SecondaryAxis></Value></Frame></Frames>  GraphicType=FromGeometry  MarkerShape=Sphere  MarkerSize=10  GraphicVisPropType=SimpleVisualProperties  GraphicDiffuseColor=[0.5 0.5 0.5]  GraphicSpecularColor=[0.5 0.5 0.5 1.0]  GraphicAmbientColor=[0.15 0.15 0.15 1.0]  GraphicEmissiveColor=[0.0 0.0 0.0 1.0]  GraphicShininess=75  GraphicOpacity=1.0
  MCP Joint : PMIOPort  Side=Left
  Head : PMIOPort  Port=2  Side=Right
  COM : PMIOPort  Port=3  Side=Right
  Base : PMIOPort  Port=4  Side=Right
  CM Joint : PMIOPort  Port=5  Side=Right
  R : PMIOPort  Port=6  Side=Right
  connections:
  CM Joint/RConn1 -- CM Joint Transform/RConn1
  MCP Joint/RConn1 -- MCP Joint Transform/RConn1
  R/RConn1 -- Rigid Body/RConn1
  MCP Joint Transform/LConn1 -- Rigid Body/LConn1 -- Base Transform/LConn1 -- CM Joint Transform/LConn1 -- COM/RConn1 -- Head Transform/LConn1
  Head/RConn1 -- Head Transform/RConn1
  Base/RConn1 -- Base Transform/RConn1

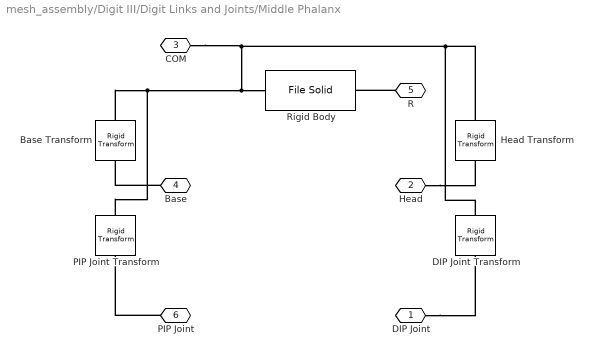
== system mesh_assembly/Digit III/Digit Links and Joints/Middle Phalanx ==
  Base Transform : sm_lib/Frames and Transforms/Rigid Transform  TranslationMethod=Cartesian  TranslationStandardOffset=0  TranslationLengthUnit=m  TranslationStandardAxis=+Z  TranslationCartesianOffset=middle_phalanx_base(1, :)  TranslationROffset=0  TranslationROffsetUnits=m  TranslationZOffset=0  TranslationZOffsetUnits=m  TranslationThetaOffset=0  TranslationThetaOffsetUnits=deg  RotationMethod=RotationSequence  RotationAngleUnits=deg  RotationStandardAxis=+Z  RotationAngle=0.0  RotationArbitraryAxis=[0 0 1]  FollAlignAxisA=+X  BaseAlignAxisA=+Y  FollAlignAxisB=+Y  BaseAlignAxisB=+Z  RotationSequenceAxes=FollowerAxes  RotationSequence=XYZ  RotationSequenceAngles=middle_phalanx_base(2, :)  RotationSequenceAnglesUnits=deg  RotationMatrix=[1 0 0; 0 1 0; 0 0 1]
  DIP Joint Transform : sm_lib/Frames and Transforms/Rigid Transform  TranslationMethod=Cartesian  TranslationStandardOffset=0  TranslationLengthUnit=m  TranslationStandardAxis=+Z  TranslationCartesianOffset=middle_phalanx_dip_joint(1, :)  TranslationROffset=0  TranslationROffsetUnits=m  TranslationZOffset=0  TranslationZOffsetUnits=m  TranslationThetaOffset=0  TranslationThetaOffsetUnits=deg  RotationMethod=RotationSequence  RotationAngleUnits=deg  RotationStandardAxis=+Z  RotationAngle=0.0  RotationArbitraryAxis=[0 0 1]  FollAlignAxisA=+X  BaseAlignAxisA=+Y  FollAlignAxisB=+Y  BaseAlignAxisB=+Z  RotationSequenceAxes=FollowerAxes  RotationSequence=XYZ  RotationSequenceAngles=middle_phalanx_dip_joint(2, :)  RotationSequenceAnglesUnits=deg  RotationMatrix=[1 0 0; 0 1 0; 0 0 1]
  Head Transform : sm_lib/Frames and Transforms/Rigid Transform  TranslationMethod=Cartesian  TranslationStandardOffset=0  TranslationLengthUnit=m  TranslationStandardAxis=+Z  TranslationCartesianOffset=middle_phalanx_head(1, :)  TranslationROffset=0  TranslationROffsetUnits=m  TranslationZOffset=0  TranslationZOffsetUnits=m  TranslationThetaOffset=0  TranslationThetaOffsetUnits=deg  RotationMethod=RotationSequence  RotationAngleUnits=deg  RotationStandardAxis=+Z  RotationAngle=0.0  RotationArbitraryAxis=[0 0 1]  FollAlignAxisA=+X  BaseAlignAxisA=+Y  FollAlignAxisB=+Y  BaseAlignAxisB=+Z  RotationSequenceAxes=FollowerAxes  RotationSequence=XYZ  RotationSequenceAngles=middle_phalanx_head(2, :)  RotationSequenceAnglesUnits=deg  RotationMatrix=[1 0 0; 0 1 0; 0 0 1]
  PIP Joint Transform : sm_lib/Frames and Transforms/Rigid Transform  TranslationMethod=Cartesian  TranslationStandardOffset=0  TranslationLengthUnit=m  TranslationStandardAxis=+Z  TranslationCartesianOffset=middle_phalanx_pip_joint(1, :)  TranslationROffset=0  TranslationROffsetUnits=m  TranslationZOffset=0  TranslationZOffsetUnits=m  TranslationThetaOffset=0  TranslationThetaOffsetUnits=deg  RotationMethod=RotationSequence  RotationAngleUnits=deg  RotationStandardAxis=+Z  RotationAngle=0.0  RotationArbitraryAxis=[0 0 1]  FollAlignAxisA=+X  BaseAlignAxisA=+Y  FollAlignAxisB=+Y  BaseAlignAxisB=+Z  RotationSequenceAxes=FollowerAxes  RotationSequence=XYZ  RotationSequenceAngles=middle_phalanx_pip_joint(2, :)  RotationSequenceAnglesUnits=deg  RotationMatrix=[1 0 0; 0 1 0; 0 0 1]
  Rigid Body : sm_lib/Body Elements/File Solid  ExtGeomFileName=C:\Users\Daniel Adejumo\Documents\MATLAB\DARM\Geometry Models and FEA\Models\Skeleton Scan\Right Hand\Digit III\Middle Phalanx III.obj  UnitType=Custom  ExtGeomFileUnits=mm  StepReaderType=HEX  ExportConvexHullGeometry=off  InertiaType=CalculateFromGeometry  Mass=1  MassUnits=kg  CenterOfMass=[0 0 0]  CenterOfMassUnits=m  MomentsOfInertia=[1 1 1]  MomentsOfInertiaUnits=kg*m^2  ProductsOfInertia=[0 0 0]  ProductsOfInertiaUnits=kg*m^2  BasedOnType=Density  Density=links_density  DensityUnits=kg/m^3  DoExposeReferenceFrame=on  SerializedFrames=<Frames><Frame><Id>Frame1</Id><Value><Name>COM</Name><Origin><Source>CenterOfMassFrame</Source><FeatureName></FeatureName></Origin><PrimaryAxis><DefinedDirection>+Z</DefinedDirection><Source>ReferenceFrame</Source><SourceDirection>+X</SourceDirection><FeatureName></FeatureName></PrimaryAxis><SecondaryAxis><DefinedDirection>+X</DefinedDirection><Source>ReferenceFrame</Source><SourceDirection>-Y</SourceDirection><FeatureName></FeatureName></SecondaryAxis></Value></Frame></Frames>  GraphicType=FromGeometry  MarkerShape=Sphere  MarkerSize=10  GraphicVisPropType=SimpleVisualProperties  GraphicDiffuseColor=[0.5 0.5 0.5]  GraphicSpecularColor=[0.5 0.5 0.5 1.0]  GraphicAmbientColor=[0.15 0.15 0.15 1.0]  GraphicEmissiveColor=[0.0 0.0 0.0 1.0]  GraphicShininess=75  GraphicOpacity=1.0
  DIP Joint : PMIOPort  Side=Left
  Head : PMIOPort  Port=2  Side=Left
  COM : PMIOPort  Port=3  Side=Left
  Base : PMIOPort  Port=4  Side=Left
  R : PMIOPort  Port=5  Side=Left
  PIP Joint : PMIOPort  Port=6  Side=Left
  connections:
  R/RConn1 -- Rigid Body/RConn1
  DIP Joint/RConn1 -- DIP Joint Transform/RConn1
  PIP Joint/RConn1 -- PIP Joint Transform/RConn1
  Head/RConn1 -- Head Transform/RConn1
  Base/RConn1 -- Base Transform/RConn1
  COM/RConn1 -- Rigid Body/LConn1 -- Base Transform/LConn1 -- PIP Joint Transform/LConn1 -- DIP Joint Transform/LConn1 -- Head Transform/LConn1

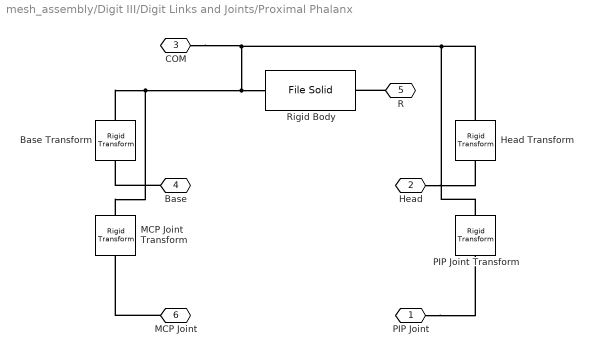
== system mesh_assembly/Digit III/Digit Links and Joints/Proximal Phalanx ==
  Base Transform : sm_lib/Frames and Transforms/Rigid Transform  TranslationMethod=Cartesian  TranslationStandardOffset=0  TranslationLengthUnit=m  TranslationStandardAxis=+Z  TranslationCartesianOffset=proximal_phalanx_base(1, :)  TranslationROffset=0  TranslationROffsetUnits=m  TranslationZOffset=0  TranslationZOffsetUnits=m  TranslationThetaOffset=0  TranslationThetaOffsetUnits=deg  RotationMethod=RotationSequence  RotationAngleUnits=deg  RotationStandardAxis=+Z  RotationAngle=0.0  RotationArbitraryAxis=[0 0 1]  FollAlignAxisA=+X  BaseAlignAxisA=+Y  FollAlignAxisB=+Y  BaseAlignAxisB=+Z  RotationSequenceAxes=FollowerAxes  RotationSequence=XYZ  RotationSequenceAngles=proximal_phalanx_base(2, :)  RotationSequenceAnglesUnits=deg  RotationMatrix=[1 0 0; 0 1 0; 0 0 1]
  Head Transform : sm_lib/Frames and Transforms/Rigid Transform  TranslationMethod=Cartesian  TranslationStandardOffset=0  TranslationLengthUnit=m  TranslationStandardAxis=+Z  TranslationCartesianOffset=proximal_phalanx_head(1, :)  TranslationROffset=0  TranslationROffsetUnits=m  TranslationZOffset=0  TranslationZOffsetUnits=m  TranslationThetaOffset=0  TranslationThetaOffsetUnits=deg  RotationMethod=RotationSequence  RotationAngleUnits=deg  RotationStandardAxis=+Z  RotationAngle=0.0  RotationArbitraryAxis=[0 0 1]  FollAlignAxisA=+X  BaseAlignAxisA=+Y  FollAlignAxisB=+Y  BaseAlignAxisB=+Z  RotationSequenceAxes=FollowerAxes  RotationSequence=XYZ  RotationSequenceAngles=proximal_phalanx_head(2, :)  RotationSequenceAnglesUnits=deg  RotationMatrix=[1 0 0; 0 1 0; 0 0 1]
  MCP Joint Transform : sm_lib/Frames and Transforms/Rigid Transform  TranslationMethod=Cartesian  TranslationStandardOffset=0  TranslationLengthUnit=m  TranslationStandardAxis=+Z  TranslationCartesianOffset=proximal_phalanx_mcp_joint(1, :)  TranslationROffset=0  TranslationROffsetUnits=m  TranslationZOffset=0  TranslationZOffsetUnits=m  TranslationThetaOffset=0  TranslationThetaOffsetUnits=deg  RotationMethod=RotationSequence  RotationAngleUnits=deg  RotationStandardAxis=+Z  RotationAngle=0.0  RotationArbitraryAxis=[0 0 1]  FollAlignAxisA=+X  BaseAlignAxisA=+Y  FollAlignAxisB=+Y  BaseAlignAxisB=+Z  RotationSequenceAxes=FollowerAxes  RotationSequence=XYZ  RotationSequenceAngles=proximal_phalanx_mcp_joint(2, :)  RotationSequenceAnglesUnits=deg  RotationMatrix=[1 0 0; 0 1 0; 0 0 1]
  PIP Joint Transform : sm_lib/Frames and Transforms/Rigid Transform  TranslationMethod=Cartesian  TranslationStandardOffset=0  TranslationLengthUnit=m  TranslationStandardAxis=+Z  TranslationCartesianOffset=proximal_phalanx_pip_joint(1, :)  TranslationROffset=0  TranslationROffsetUnits=m  TranslationZOffset=0  TranslationZOffsetUnits=m  TranslationThetaOffset=0  TranslationThetaOffsetUnits=deg  RotationMethod=RotationSequence  RotationAngleUnits=deg  RotationStandardAxis=+Z  RotationAngle=0.0  RotationArbitraryAxis=[0 0 1]  FollAlignAxisA=+X  BaseAlignAxisA=+Y  FollAlignAxisB=+Y  BaseAlignAxisB=+Z  RotationSequenceAxes=FollowerAxes  RotationSequence=XYZ  RotationSequenceAngles=proximal_phalanx_pip_joint(2, :)  RotationSequenceAnglesUnits=deg  RotationMatrix=[1 0 0; 0 1 0; 0 0 1]
  Rigid Body : sm_lib/Body Elements/File Solid  ExtGeomFileName=C:\Users\Daniel Adejumo\Documents\MATLAB\DARM\Geometry Models and FEA\Models\Skeleton Scan\Right Hand\Digit III\Proximal Phalanx III.obj  UnitType=Custom  ExtGeomFileUnits=mm  StepReaderType=HEX  ExportConvexHullGeometry=off  InertiaType=CalculateFromGeometry  Mass=1  MassUnits=kg  CenterOfMass=[0 0 0]  CenterOfMassUnits=m  MomentsOfInertia=[1 1 1]  MomentsOfInertiaUnits=kg*m^2  ProductsOfInertia=[0 0 0]  ProductsOfInertiaUnits=kg*m^2  BasedOnType=Density  Density=links_density  DensityUnits=kg/m^3  DoExposeReferenceFrame=on  SerializedFrames=<Frames><Frame><Id>Frame1</Id><Value><Name>COM</Name><Origin><Source>CenterOfMassFrame</Source><FeatureName></FeatureName></Origin><PrimaryAxis><DefinedDirection>+Z</DefinedDirection><Source>ReferenceFrame</Source><SourceDirection>-Z</SourceDirection><FeatureName></FeatureName></PrimaryAxis><SecondaryAxis><DefinedDirection>+X</DefinedDirection><Source>ReferenceFrame</Source><SourceDirection>-Y</SourceDirection><FeatureName></FeatureName></SecondaryAxis></Value></Frame></Frames>  GraphicType=FromGeometry  MarkerShape=Sphere  MarkerSize=10  GraphicVisPropType=SimpleVisualProperties  GraphicDiffuseColor=[0.5 0.5 0.5]  GraphicSpecularColor=[0.5 0.5 0.5 1.0]  GraphicAmbientColor=[0.15 0.15 0.15 1.0]  GraphicEmissiveColor=[0.0 0.0 0.0 1.0]  GraphicShininess=75  GraphicOpacity=1.0
  PIP Joint : PMIOPort  Side=Left
  Head : PMIOPort  Port=2  Side=Left
  COM : PMIOPort  Port=3  Side=Left
  Base : PMIOPort  Port=4  Side=Left
  R : PMIOPort  Port=5  Side=Left
  MCP Joint : PMIOPort  Port=6  Side=Right
  connections:
  R/RConn1 -- Rigid Body/RConn1
  MCP Joint/RConn1 -- MCP Joint Transform/RConn1
  PIP Joint/RConn1 -- PIP Joint Transform/RConn1
  Base/RConn1 -- Base Transform/RConn1
  COM/RConn1 -- Rigid Body/LConn1 -- Base Transform/LConn1 -- MCP Joint Transform/LConn1 -- PIP Joint Transform/LConn1 -- Head Transform/LConn1
  Head/RConn1 -- Head Transform/RConn1

== system mesh_assembly/Digit IV/Digit Links and Joints/Distal Phalanx ==
  Base Transform : sm_lib/Frames and Transforms/Rigid Transform  TranslationMethod=Cartesian  TranslationStandardOffset=0  TranslationLengthUnit=m  TranslationStandardAxis=+Z  TranslationCartesianOffset=distal_phalanx_base(1, :)  TranslationROffset=0  TranslationROffsetUnits=m  TranslationZOffset=0  TranslationZOffsetUnits=m  TranslationThetaOffset=0  TranslationThetaOffsetUnits=deg  RotationMethod=RotationSequence  RotationAngleUnits=deg  RotationStandardAxis=+Z  RotationAngle=0.0  RotationArbitraryAxis=[0 0 1]  FollAlignAxisA=+X  BaseAlignAxisA=+Y  FollAlignAxisB=+Y  BaseAlignAxisB=+Z  RotationSequenceAxes=FollowerAxes  RotationSequence=XYZ  RotationSequenceAngles=distal_phalanx_base(2, :)  RotationSequenceAnglesUnits=deg  RotationMatrix=[1 0 0; 0 1 0; 0 0 1]
  DIP Joint Transform : sm_lib/Frames and Transforms/Rigid Transform  TranslationMethod=Cartesian  TranslationStandardOffset=0  TranslationLengthUnit=m  TranslationStandardAxis=+Z  TranslationCartesianOffset=distal_phalanx_dip_joint(1, :)  TranslationROffset=0  TranslationROffsetUnits=m  TranslationZOffset=0  TranslationZOffsetUnits=m  TranslationThetaOffset=0  TranslationThetaOffsetUnits=deg  RotationMethod=RotationSequence  RotationAngleUnits=deg  RotationStandardAxis=+Z  RotationAngle=0.0  RotationArbitraryAxis=[0 0 1]  FollAlignAxisA=+X  BaseAlignAxisA=+Y  FollAlignAxisB=+Y  BaseAlignAxisB=+Z  RotationSequenceAxes=FollowerAxes  RotationSequence=XYZ  RotationSequenceAngles=distal_phalanx_dip_joint(2, :)  RotationSequenceAnglesUnits=deg  RotationMatrix=[1 0 0; 0 1 0; 0 0 1]
  Head Transform : sm_lib/Frames and Transforms/Rigid Transform  TranslationMethod=Cartesian  TranslationStandardOffset=0  TranslationLengthUnit=m  TranslationStandardAxis=+Z  TranslationCartesianOffset=distal_phalanx_head(1, :)  TranslationROffset=0  TranslationROffsetUnits=m  TranslationZOffset=0  TranslationZOffsetUnits=m  TranslationThetaOffset=0  TranslationThetaOffsetUnits=deg  RotationMethod=RotationSequence  RotationAngleUnits=deg  RotationStandardAxis=+Z  RotationAngle=0.0  RotationArbitraryAxis=[0 0 1]  FollAlignAxisA=+X  BaseAlignAxisA=+Y  FollAlignAxisB=+Y  BaseAlignAxisB=+Z  RotationSequenceAxes=FollowerAxes  RotationSequence=XYZ  RotationSequenceAngles=distal_phalanx_head(2, :)  RotationSequenceAnglesUnits=deg  RotationMatrix=[1 0 0; 0 1 0; 0 0 1]
  Rigid Body : sm_lib/Body Elements/File Solid  ExtGeomFileName=C:\Users\Daniel Adejumo\Documents\MATLAB\DARM\Geometry Models and FEA\Models\Skeleton Scan\Right Hand\Digit IV\Distal Phalanx IV.obj  UnitType=Custom  ExtGeomFileUnits=mm  StepReaderType=HEX  ExportConvexHullGeometry=off  InertiaType=CalculateFromGeometry  Mass=1  MassUnits=kg  CenterOfMass=[0 0 0]  CenterOfMassUnits=m  MomentsOfInertia=[1 1 1]  MomentsOfInertiaUnits=kg*m^2  ProductsOfInertia=[0 0 0]  ProductsOfInertiaUnits=kg*m^2  BasedOnType=Density  Density=links_density  DensityUnits=kg/m^3  DoExposeReferenceFrame=on  SerializedFrames=<Frames><Frame><Id>Frame1</Id><Value><Name>COM</Name><Origin><Source>CenterOfMassFrame</Source><FeatureName></FeatureName></Origin><PrimaryAxis><DefinedDirection>+Z</DefinedDirection><Source>ReferenceFrame</Source><SourceDirection>+X</SourceDirection><FeatureName></FeatureName></PrimaryAxis><SecondaryAxis><DefinedDirection>+X</DefinedDirection><Source>ReferenceFrame</Source><SourceDirection>-Y</SourceDirection><FeatureName></FeatureName></SecondaryAxis></Value></Frame></Frames>  GraphicType=FromGeometry  MarkerShape=Sphere  MarkerSize=10  GraphicVisPropType=SimpleVisualProperties  GraphicDiffuseColor=[0.5 0.5 0.5]  GraphicSpecularColor=[0.5 0.5 0.5 1.0]  GraphicAmbientColor=[0.15 0.15 0.15 1.0]  GraphicEmissiveColor=[0.0 0.0 0.0 1.0]  GraphicShininess=75  GraphicOpacity=1.0
  Head : PMIOPort  Side=Left
  COM : PMIOPort  Port=2  Side=Left
  Base : PMIOPort  Port=3  Side=Left
  R : PMIOPort  Port=4  Side=Left
  DIP Joint : PMIOPort  Port=5  Side=Left
  connections:
  R/RConn1 -- Rigid Body/RConn1
  Head/RConn1 -- Head Transform/RConn1
  DIP Joint/RConn1 -- DIP Joint Transform/RConn1
  Base/RConn1 -- Base Transform/RConn1
  DIP Joint Transform/LConn1 -- Rigid Body/LConn1 -- Head Transform/LConn1 -- COM/RConn1 -- Base Transform/LConn1
